simulink model "SistemaMasaResorteAmortiguador"  (R2019a)
settings: Solver=VariableStepAuto  StartTime=0.0  StopTime=50  RelTol=1e-3
settings Model: Creator=User  LastModifiedBy=User

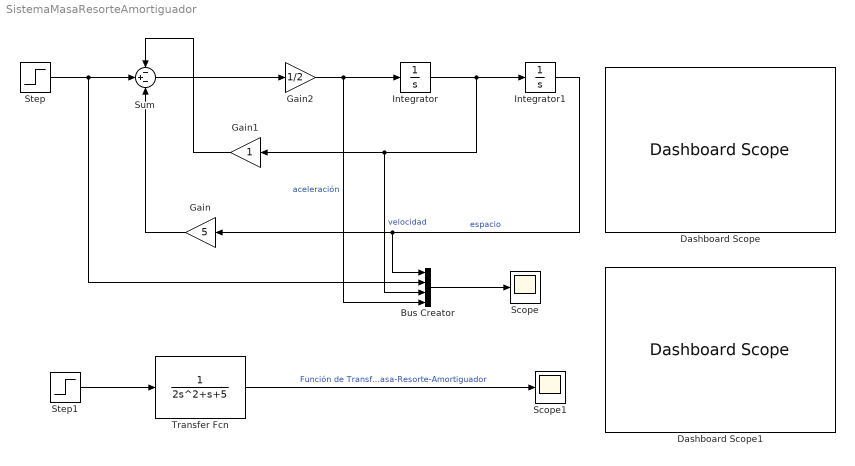
== system SistemaMasaResorteAmortiguador ==
  Bus Creator : BusCreator  Inputs=4
  Dashboard Scope : DashboardScope
  Dashboard Scope1 : DashboardScope
  Gain : Gain  Gain=5
  Gain1 : Gain
  Gain2 : Gain  Gain=1/2
  Integrator : Integrator
  Integrator1 : Integrator
  Scope : Scope
  Scope1 : Scope
  Step : Step  SampleTime=0
  Step1 : Step  SampleTime=0
  Sum : Sum  Inputs=-+-
  Transfer Fcn : TransferFcn  Denominator=[2 1 5]
  wires:
  Step/1 -> Bus Creator/2, Sum/2
  Gain/1 -> Sum/3
  Gain1/1 -> Sum/1
  Sum/1 -> Gain2/1
  Gain2/1 -> Bus Creator/4, Integrator/1  "aceleración"
  Integrator/1 -> Bus Creator/3, Gain1/1, Integrator1/1  "velocidad"
  Integrator1/1 -> Bus Creator/1, Gain/1  "espacio"
  Bus Creator/1 -> Scope/1
  Transfer Fcn/1 -> Scope1/1  "Función de Transferencia Sistema Masa-Resorte-Amortiguador"
  Step1/1 -> Transfer Fcn/1
